simulink model "final_integration_BLDC_motor"  (R2020b)
settings: Solver=VariableStepAuto  StartTime=0.0  StopTime=10.0  RelTol=1e-3
settings Model: Creator=omkar  LastModifiedBy=omkar

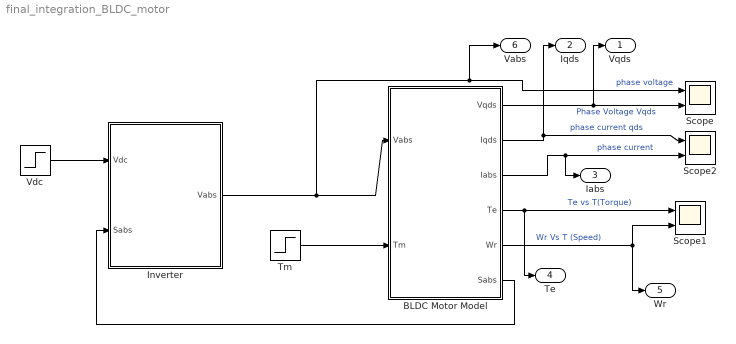
== system final_integration_BLDC_motor ==
  BLDC Motor Model : Subsystem  mask{Tm=3.53e-3, J=2.12e-6, Dm=6.04e-6, Lss=10.1e-3, rs=5.2, Lam=1.65e-2, Ts=0.001942307692308, P=4}
      mask prompts: Tm "Tm [in N m]"; J "J [in kg m^2]"; Dm "Dm [in N.m.s]"; Lss "Lss [ in H]"; rs "rs [in Ohms]"; Lam "Lam [in V*s/rad]"; Ts "Ts = Lss/rs"; P "P [no of poles]"
  Inverter : Subsystem
  Scope : Scope  NumInputPorts=2
  Scope1 : Scope  NumInputPorts=2
  Scope2 : Scope  NumInputPorts=2
  Tm : Step  Time=0.5  After=3.53e-3  SampleTime=0
  Vdc : Step  Time=0.05  After=6  SampleTime=0
  Vqds : Outport
  Iqds : Outport  Port=2
  Iabs : Outport  Port=3
  Te : Outport  Port=4
  Wr : Outport  Port=5
  Vabs : Outport  Port=6
  wires:
  BLDC Motor Model/1(Vqds) -> Scope/2, Vqds/1  "Phase Voltage Vqds"
  BLDC Motor Model/4(Te) -> Scope1/1, Te/1  "Te vs T(Torque)"
  Vdc/1 -> Inverter/1(Vdc)
  Tm/1 -> BLDC Motor Model/2(Tm)
  BLDC Motor Model/6(Sabs) -> Inverter/2(Sabs)
  BLDC Motor Model/2(Iqds) -> Iqds/1, Scope2/1  "phase current qds"
  BLDC Motor Model/3(Iabs) -> Scope2/2, Iabs/1  "phase current"
  BLDC Motor Model/5(Wr) -> Wr/1, Scope1/2  "Wr Vs T (Speed)"
  Inverter/1(Vabs) -> Scope/1, Vabs/1, BLDC Motor Model/1(Vabs)  "phase voltage"

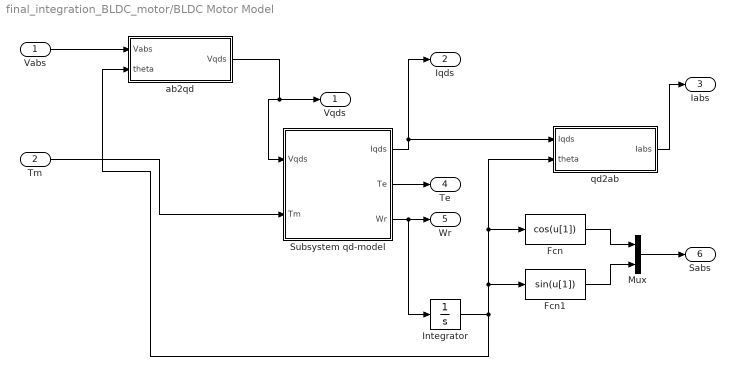
== system final_integration_BLDC_motor/BLDC Motor Model ==
  Vabs : Inport
  Tm : Inport  Port=2
  Fcn : Fcn  Expr=cos(u[1])
  Fcn1 : Fcn
  Integrator : Integrator
  Mux : Mux  Inputs=2
  Subsystem qd-model : Subsystem
  ab2qd : Subsystem
  qd2ab : Subsystem
  Vqds : Outport
  Iqds : Outport  Port=2
  Iabs : Outport  Port=3
  Te : Outport  Port=4
  Wr : Outport  Port=5
  Sabs : Outport  Port=6
  wires:
  Vabs/1 -> ab2qd/1(Vabs)
  ab2qd/1(" Vqds") -> Subsystem qd-model/1(Vqds), Vqds/1
  Tm/1 -> Subsystem qd-model/2(Tm)
  Subsystem qd-model/1(Iqds) -> Iqds/1, qd2ab/1(Iqds)
  qd2ab/1(" Iabs") -> Iabs/1
  Subsystem qd-model/2(Te) -> Te/1
  Subsystem qd-model/3(Wr) -> Integrator/1, Wr/1
  Integrator/1 -> ab2qd/2(theta), Fcn1/1, qd2ab/2(theta), Fcn/1
  Mux/1 -> Sabs/1
  Fcn/1 -> Mux/1
  Fcn1/1 -> Mux/2

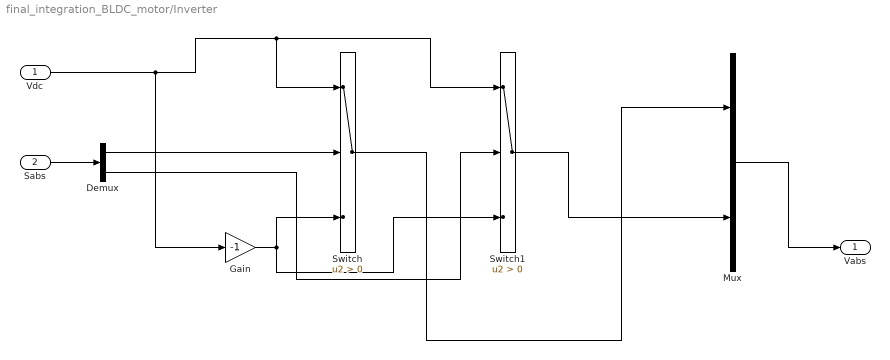
== system final_integration_BLDC_motor/Inverter ==
  Vdc : Inport
  Sabs : Inport  Port=2
  Demux : Demux  Outputs=2
  Gain : Gain  Gain=-1
  Mux : Mux  Inputs=2
  Switch : Switch  Criteria=u2 > Threshold
  Switch1 : Switch  Criteria=u2 > Threshold
  Vabs : Outport
  wires:
  Sabs/1 -> Demux/1
  Mux/1 -> Vabs/1
  Demux/1 -> Switch/2
  Vdc/1 -> Gain/1, Switch/1, Switch1/1
  Switch/1 -> Mux/1
  Switch1/1 -> Mux/2
  Demux/2 -> Switch1/2
  Gain/1 -> Switch/3, Switch1/3

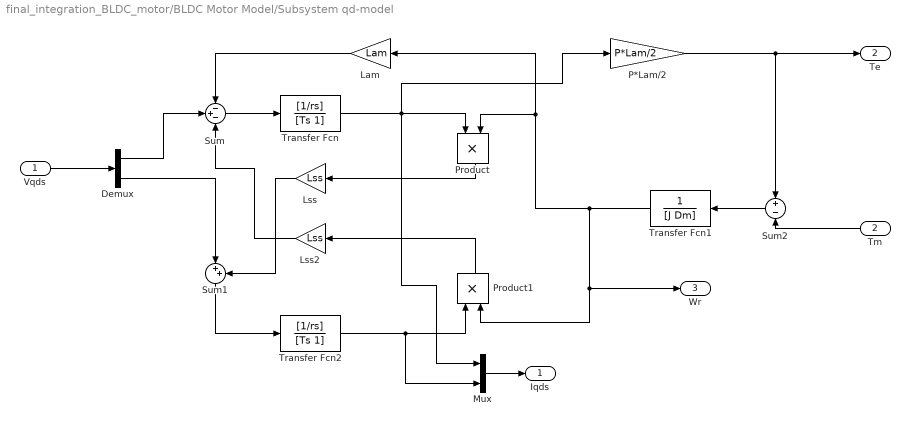
== system final_integration_BLDC_motor/BLDC Motor Model/Subsystem qd-model ==
  Vqds : Inport
  Tm : Inport  Port=2
  Demux : Demux  Outputs=2
  Lam : Gain  Gain=Lam
  Lss : Gain  Gain=Lss
  Lss2 : Gain  Gain=Lss
  Mux : Mux  Inputs=2
  P*Lam/2 : Gain  Gain=P*Lam/2
  Product : Product
  Product1 : Product
  Sum : Sum  Inputs=-+-
  Sum1 : Sum  Inputs=|++
  Sum2 : Sum  Inputs=+-
  Transfer Fcn : TransferFcn  Numerator=[1/rs]  Denominator=[Ts 1]
  Transfer Fcn1 : TransferFcn  Denominator=[J Dm]
  Transfer Fcn2 : TransferFcn  Numerator=[1/rs]  Denominator=[Ts 1]
  Iqds : Outport
  Te : Outport  Port=2
  Wr : Outport  Port=3
  wires:
  Vqds/1 -> Demux/1
  Demux/1 -> Sum/2
  Demux/2 -> Sum1/1
  P*Lam/2/1 -> Sum2/1, Te/1
  Tm/1 -> Sum2/2
  Sum/1 -> Transfer Fcn/1
  Lam/1 -> Sum/1
  Lss2/1 -> Sum/3
  Lss/1 -> Sum1/2
  Sum1/1 -> Transfer Fcn2/1
  Sum2/1 -> Transfer Fcn1/1
  Transfer Fcn2/1 -> Mux/2, Product1/1
  Product1/1 -> Lss2/1
  Product/1 -> Lss/1
  Transfer Fcn/1 -> Mux/1, P*Lam/2/1, Product/1
  Transfer Fcn1/1 -> Product/2, Lam/1, Product1/2, Wr/1
  Mux/1 -> Iqds/1

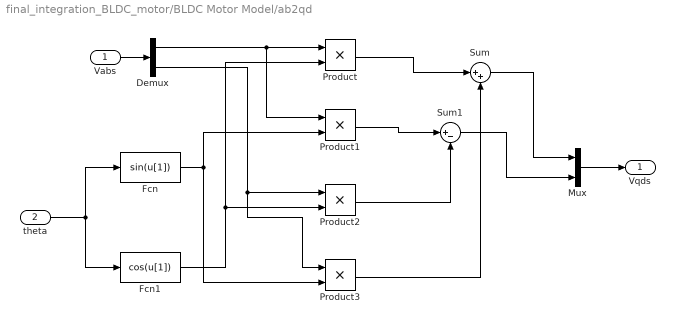
== system final_integration_BLDC_motor/BLDC Motor Model/ab2qd ==
  Vabs : Inport
  theta : Inport  Port=2
  Demux : Demux  Outputs=2
  Fcn : Fcn
  Fcn1 : Fcn  Expr=cos(u[1])
  Mux : Mux  Inputs=2
  Product{,1..3} (4 alike) : Product
  Sum : Sum  Inputs=|++
  Sum1 : Sum  Inputs=|+-
  " Vqds" : Outport
  wires:
  Vabs/1 -> Demux/1
  Mux/1 -> " Vqds"/1
  theta/1 -> Fcn/1, Fcn1/1
  Demux/1 -> Product1/1, Product/1
  Fcn1/1 -> Product2/2, Product/2
  Fcn/1 -> Product1/2, Product3/2
  Demux/2 -> Product3/1, Product2/1
  Product/1 -> Sum/1
  Product3/1 -> Sum/2
  Sum/1 -> Mux/1
  Product1/1 -> Sum1/1
  Product2/1 -> Sum1/2
  Sum1/1 -> Mux/2

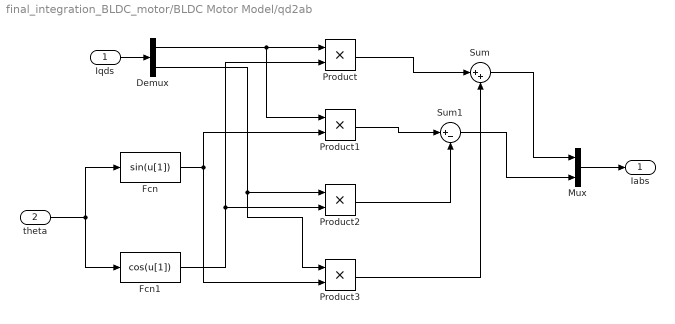
== system final_integration_BLDC_motor/BLDC Motor Model/qd2ab ==
  Iqds : Inport
  theta : Inport  Port=2
  Demux : Demux  Outputs=2
  Fcn : Fcn
  Fcn1 : Fcn  Expr=cos(u[1])
  Mux : Mux  Inputs=2
  Product{,1..3} (4 alike) : Product
  Sum : Sum  Inputs=|++
  Sum1 : Sum  Inputs=|+-
  " Iabs" : Outport
  wires:
  Iqds/1 -> Demux/1
  Mux/1 -> " Iabs"/1
  theta/1 -> Fcn/1, Fcn1/1
  Demux/1 -> Product1/1, Product/1
  Fcn1/1 -> Product2/2, Product/2
  Fcn/1 -> Product1/2, Product3/2
  Demux/2 -> Product3/1, Product2/1
  Product/1 -> Sum/1
  Product3/1 -> Sum/2
  Sum/1 -> Mux/1
  Product1/1 -> Sum1/1
  Product2/1 -> Sum1/2
  Sum1/1 -> Mux/2
